simulink model "ap3_main"  (R2021b)
settings: Solver=ode45  StartTime=0.0  StopTime=30  MaxStep=0.01  RelTol=1e-3
settings Model: Creator=Usuario_UMA  LastModifiedBy=Daniel
settings SolverCC: AlgebraicLoopSolver=TrustRegion
settings DebuggingCC: SFMachineParentedDataDiag=warning

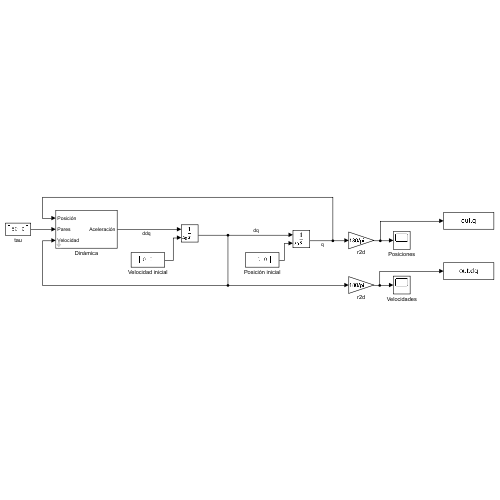
[thumbnail: Simulink's stored preview of the top-level diagram]
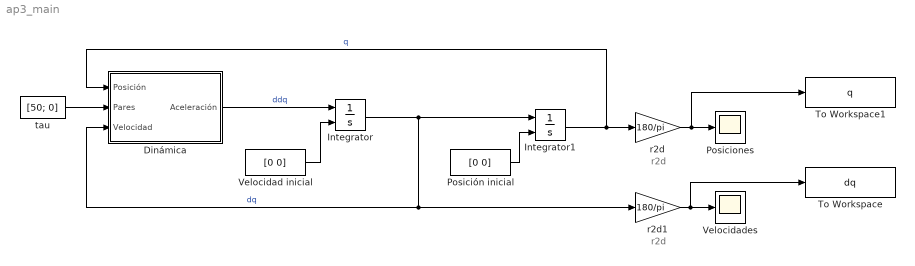
== system ap3_main ==
  note: r2d
  note: r2d
  Dinámica : Subsystem  mask{m1=5, l1=1, m2=2, l2=0.6, fv1=4.5, fv2=3.5}
      mask prompts: m1 "Masa de art. 1 (kg)"; l1 "Longitud de art. 1 (m)"; m2 "Masa de art. 2 (kg)"; l2 "Longitud de art. 2 (m)"; fv1 "Coeficiente fricción de art. 1"; fv2 "Coeficiente fricción de art. 2"
  Integrator : Integrator  InitialConditionSource=external
  Integrator1 : Integrator  InitialConditionSource=external
  Posiciones : Scope
  Posición inicial : Constant  Value=[0 0]
  To Workspace : ToWorkspace  VariableName=dq  SampleTime=-1
      settings: Save2DSignal=2-D array (concatenate along first dimension)
  To Workspace1 : ToWorkspace  VariableName=q  SampleTime=-1
      settings: Save2DSignal=2-D array (concatenate along first dimension)
  Velocidad inicial : Constant  Value=[0 0]
  Velocidades : Scope
  r2d : Gain  Gain=180/pi
  r2d1 : Gain  Gain=180/pi
  tau : Constant  Value=[50; 0]
  wires:
  Integrator/1 -> Integrator1/1, Dinámica/3(Velocidad), r2d1/1  "dq"
  Velocidad inicial/1 -> Integrator/2
  Posición inicial/1 -> Integrator1/2
  Integrator1/1 -> Dinámica/1(Posición), r2d/1  "q"
  Dinámica/1(Aceleración) -> Integrator/1  "ddq"
  tau/1 -> Dinámica/2(Pares)
  r2d/1 -> To Workspace1/1, Posiciones/1
  r2d1/1 -> To Workspace/1, Velocidades/1

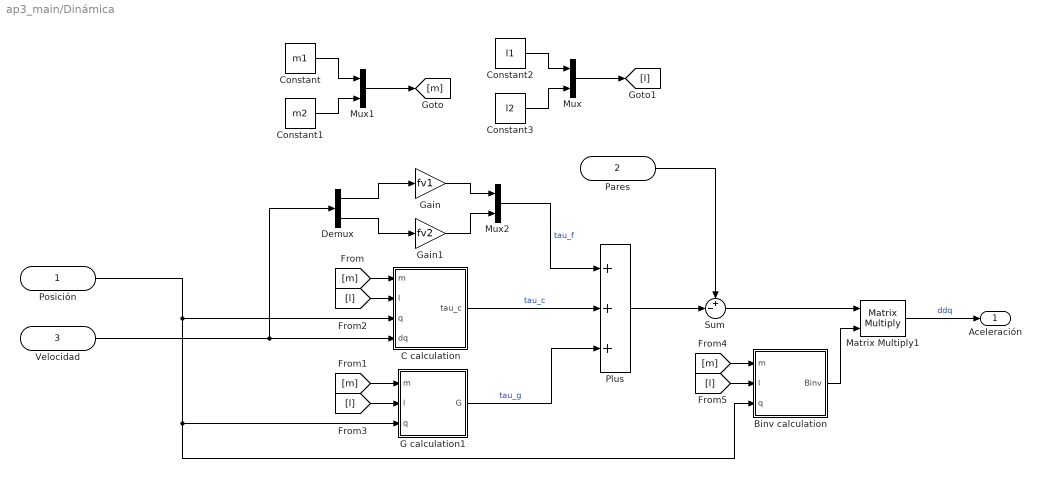
== system ap3_main/Dinámica ==
  Posición : Inport
  Pares : Inport  Port=2
  Velocidad : Inport  Port=3
  Binv calculation : MATLAB Function  TreatAsAtomicUnit=on
  C calculation : MATLAB Function  TreatAsAtomicUnit=on
  Constant : Constant  Value=m1
  Constant1 : Constant  Value=m2
  Constant2 : Constant  Value=l1
  Constant3 : Constant  Value=l2
  Demux : Demux  Outputs=2
  G calculation1 : MATLAB Function  TreatAsAtomicUnit=on
  Gain : Gain  Gain=fv1
  Gain1 : Gain  Gain=fv2
  Matrix Multiply1 : Product  Multiplication=Matrix(*)
  Mux : Mux  Inputs=2
  Mux1 : Mux  Inputs=2
  Mux2 : Mux  Inputs=2
  Plus : Sum  Inputs=+++
  Sum : Sum  Inputs=+-|
  Aceleración : Outport
  wires:
  Constant2/1 -> Mux/1
  Constant3/1 -> Mux/2
  Constant/1 -> Mux1/1
  Constant1/1 -> Mux1/2
  Mux/1 -> [l]
  Posición/1 -> Binv calculation/3(q), G calculation1/3(q), C calculation/3(q)
  Mux1/1 -> [m]
  C calculation/1(tau_c) -> Plus/2  "tau_c"
  G calculation1/1(G) -> Plus/3  "tau_g"
  Pares/1 -> Sum/1
  Plus/1 -> Sum/2
  Sum/1 -> Matrix Multiply1/1
  Binv calculation/1(Binv) -> Matrix Multiply1/2
  Matrix Multiply1/1 -> Aceleración/1  "ddq"
  Velocidad/1 -> Demux/1, C calculation/4(dq)
  Demux/1 -> Gain/1
  Demux/2 -> Gain1/1
  Gain/1 -> Mux2/1
  Gain1/1 -> Mux2/2
  Mux2/1 -> Plus/1  "tau_f"
  [m] -> C calculation/1(m)
  [m] -> G calculation1/1(m)
  [l] -> C calculation/2(l)
  [l] -> G calculation1/2(l)
  [m] -> Binv calculation/1(m)
  [l] -> Binv calculation/2(l)

== matlab function ap3_main/Dinámica/C calculation ==
  data: m input; tau_c output; l input; q input; dq input
function tau_c = fcn(m,l,q,dq)

tau_c = zeros(2,1);

c=cos(q); s=sin(q); c12=cos(q(1)+q(2));

tau_c(1,1) = -m(2)*l(2)*l(1)*s(2)*(2*dq(1)+dq(2))*dq(2);
tau_c(2,1) = dq(1)^2*m(2)*l(2)*l(1)*s(2);

end

== matlab function ap3_main/Dinámica/Binv calculation ==
  data: m input; Binv output; l input; q input
function Binv = fcn(m,l,q)

B = zeros(2);

c=cos(q); s=sin(q); c12=cos(q(1)+q(2));

B(1,1) = m(1)*l(1)^2 + m(2)*l(1)^2 + 2*m(2)*l(1)*l(2)*c(2) + m(2)*l(2)^2;
B(1,2) = m(2)*l(2)^2 + m(2)*l(2)*l(1)*c(2);
B(2,1) = m(2)*l(2)^2 + m(2)*l(2)*l(1)*c(2);
B(2,2) = m(2)*l(2)^2;

Binv = inv(B);

end

== matlab function ap3_main/Dinámica/G calculation1 ==
  data: m input; G output; l input; q input
function G = fcn(m,l,q)

G = zeros(2,1);
g = 9.8;

c=cos(q); s=sin(q); c12=cos(q(1)+q(2));

G(1,1) = m(1)*g*c(1)*l(1)+m(2)*g*(c12*l(2)+c(1)*l(1));
G(2,1) = m(2)*g*c12*l(2);

end
